simulink model "ODrive_test"  (R2018b)
settings: Solver=FixedStepAuto  StartTime=0.0  StopTime=5  FixedStep=1/50  RelTol=1e-3  EnableMultiTasking=on
libraries: raspi_drivers x1
settings Model: SimulationMode=external  Creator=marti  LastModifiedBy=marti
settings SolverCC: PositivePriorityOrder=on
settings OptimizationCC: EnhancedBackFolding=on  PassReuseOutputArgsAs=Individual arguments  MaxStackSize=64  OptimizeBlockOrder=speed  DifferentSizesBufferReuse=on  OptimizationCustomize=off
settings DebuggingCC: ParameterTunabilityLossMsg=error
settings HardwareCC: ProdBitPerPointer=32  ProdBitPerSizeT=32  ProdBitPerPtrDiffT=32  ProdLargestAtomicInteger=Long  ProdLargestAtomicFloat=Double  ProdWordSize=32  ProdHWDeviceType=ARM Compatible->ARM Cortex
settings SFSimCC: MATLABDynamicMemAlloc=off
settings RTWCC: SystemTargetFile=ert.tlc  HardwareBoard=Raspberry Pi  TLCOptions="-aInlineSetEventsForThisBaseRateFcn=TLC_FALSE -aSuppressMultiTaskScheduler=TLC_FALSE  -aRateBasedStepFcn=0"  TemplateMakefile=ert_default_tmf  GenerateReport=on  Toolchain=GNU GCC Raspberry Pi  BuildConfiguration=Faster Runs  IncludeHyperlinkInReport=on  LaunchReport=on  GenerateTraceInfo=on  GenerateTraceReport=on  GenerateTraceReportSl=on  GenerateTraceReportSf=on  GenerateTraceReportEml=on
settings CodeAppCC: ForceParamTrailComments=on  IgnoreCustomStorageClasses=off  OperatorAnnotations=on  SimulinkDataObjDesc=on  SFDataObjDesc=on  InsertBlockDesc=on
settings ERTTargetCC: SupportVariableSizeSignals=on

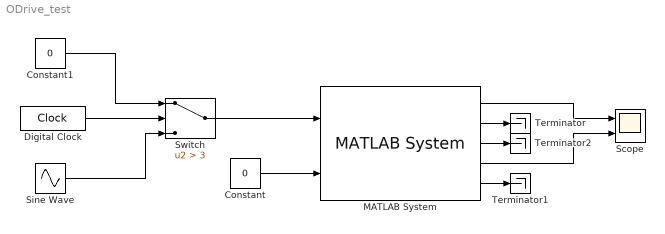
== system ODrive_test ==
  Constant : Constant  Value=0
  Constant1 : Constant  Value=0
  Digital Clock : DigitalClock  SampleTime=-1
  MATLAB System : raspi_drivers/Subsystem/MATLAB System  Maxcurrent=50  Vel_limit=50000  Control_mode=current  Motor0=on  Motor1=off  Setup_done=on  Extra_read=on
  Scope : Scope  NumInputPorts=2
  Sine Wave : Sin  Amplitude=3  Frequency=2*pi/0.7
  Switch : Switch  Criteria=u2 > Threshold  Threshold=3
  Terminator : Terminator
  Terminator1 : Terminator
  Terminator2 : Terminator
  wires:
  MATLAB System/2 -> Terminator/1
  MATLAB System/5 -> Terminator1/1
  MATLAB System/3 -> Terminator2/1
  Constant/1 -> MATLAB System/2
  MATLAB System/1 -> Scope/1
  MATLAB System/4 -> Scope/2
  Switch/1 -> MATLAB System/1
  Digital Clock/1 -> Switch/2
  Constant1/1 -> Switch/1
  Sine Wave/1 -> Switch/3
